simulink model "lookup_nD_TestGen8"  (R2017b)
settings: Solver=FixedStepDiscrete  StartTime=0.0  StopTime=10.0  RelTol=1e-3
undefined symbols (not defined in the file): Block_TestLib, reset
settings Model: Creator=ktrinh  LastModifiedBy=ktrinh
settings DebuggingCC: ParameterOverflowMsg=none

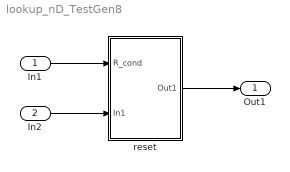
== system lookup_nD_TestGen8 ==
  In1 : Inport
  In2 : Inport  Port=2
  reset : Subsystem  AncestorBlock=Block_TestLib/reset
  Out1 : Outport
  wires:
  In1/1 -> reset/1(R_cond)
  In2/1 -> reset/2(In1)
  reset/1(Out1) -> Out1/1

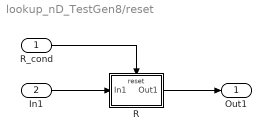
== system lookup_nD_TestGen8/reset ==
  R_cond : Inport  OutDataTypeStr=boolean
  In1 : Inport  Port=2
  R : Subsystem  TreatAsAtomicUnit=on
  Out1 : Outport
  wires:
  R_cond/1 -> R/Reset
  In1/1 -> R/1(In1)
  R/1(Out1) -> Out1/1

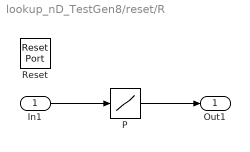
== system lookup_nD_TestGen8/reset/R ==
  In1 : Inport  PortDimensions=2
  Reset : ResetPort  DisableCoverage=on
  P : Lookup_n-D  BreakpointsSpecification=Even spacing  BreakpointsForDimension3=[5, 7]  BreakpointsForDimension1FirstPoint=52.0861  BreakpointsForDimension2FirstPoint=108.8669  BreakpointsForDimension1Spacing=1.5  BreakpointsForDimension2Spacing=1.5  UseOneInputPortForAllInputData=on  Table=[72.2105693536706 113.872127169376 52.585196284929 74.362227336977 122.993394096973;19.4123549104279 85.7057277634569 83.2562213177174 103.093323114898 36.839766420793;85.169505633284 83.5595624264661 50.5502755470171 86.5962887367263 2.00006489747968]  InterpMethod=Flat  UseLastTableValue=on  InternalRulePriority=Speed  RndMeth=Simplest  InputSameDT=on
  Out1 : Outport
  wires:
  In1/1 -> P/1
  P/1 -> Out1/1
